simulink model "pendulum_model"  (R2025b)
settings: Solver=FixedStepAuto  StartTime=0.0  StopTime=10.0  RelTol=1e-3
values from neighbouring files (symbols this model uses):
  a = max(a, 0)    [forward_agent.m]
undefined symbols (not defined in the file or in its folder): b, c, d, Km, x0
settings Model: Creator=filip  LastModifiedBy=filip
settings ModelReferenceCC: ModelReferenceMinAlgLoopOccurrences=on

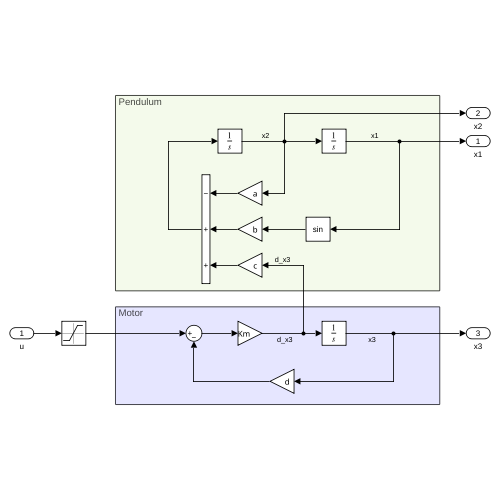
[thumbnail: Simulink's stored preview of the top-level diagram]
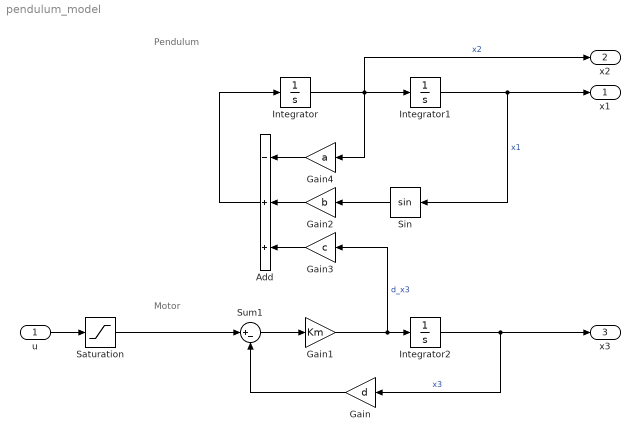
== system pendulum_model ==
  note: Pendulum
  note: Motor
  u : Inport
  Add : Sum  Inputs=-++
  Gain : Gain  Gain=d
  Gain1 : Gain  Gain=Km
  Gain2 : Gain  Gain=b
  Gain3 : Gain  Gain=c
  Gain4 : Gain  Gain=a
  Integrator : Integrator  InitialCondition=x0(2)
  Integrator1 : Integrator  InitialCondition=x0(1)
  Integrator2 : Integrator  InitialCondition=x0(3)
  Saturation : Saturate  UpperLimit=1  LowerLimit=-1
  Sin : Trigonometry
  Sum1 : Sum  Inputs=|+-
  x1 : Outport
  x2 : Outport  Port=2
  x3 : Outport  Port=3
  wires:
  Gain3/1 -> Add/3
  Saturation/1 -> Sum1/1
  u/1 -> Saturation/1
  Integrator2/1 -> x3/1, Gain/1  "x3"
  Gain1/1 -> Gain3/1, Integrator2/1  "d_x3"
  Integrator1/1 -> x1/1, Sin/1  "x1"
  Integrator/1 -> x2/1, Integrator1/1, Gain4/1  "x2"
  Sum1/1 -> Gain1/1
  Gain2/1 -> Add/2
  Sin/1 -> Gain2/1
  Gain4/1 -> Add/1
  Gain/1 -> Sum1/2
  Add/1 -> Integrator/1
